simulink model "Slx002_M1_TTRobot"  (R2017b)
settings: Solver=FixedStepAuto  StartTime=0  StopTime=100.0  FixedStep=0.001  RelTol=1e-3
settings Model: Creator=Dell  LastModifiedBy=Dell

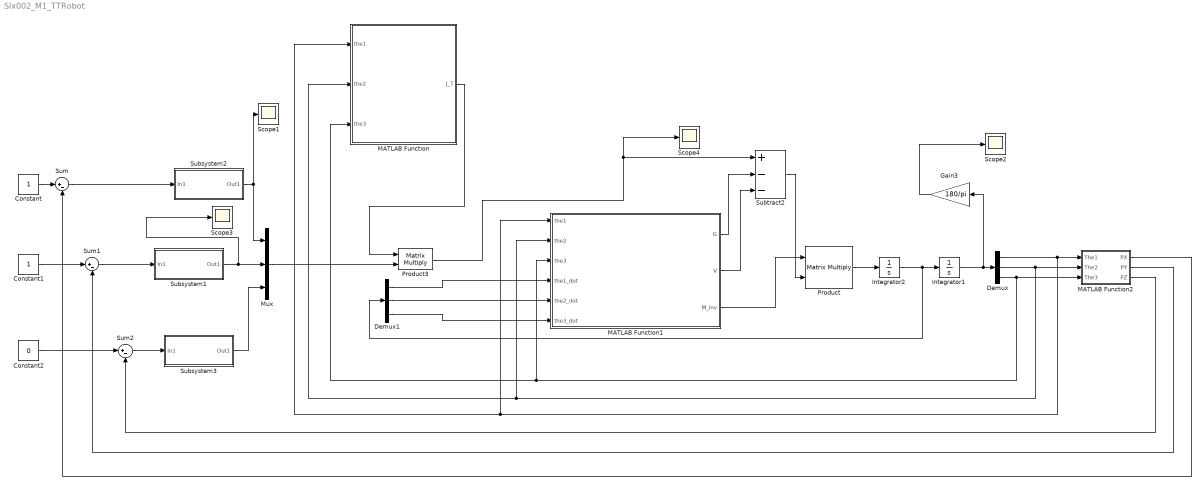
== system Slx002_M1_TTRobot ==
  Constant : Constant
  Constant1 : Constant
  Constant2 : Constant  Value=0
  Demux : Demux  Outputs=3
  Demux1 : Demux  Outputs=3
  Gain3 : Gain  Gain=180/pi
  Integrator1 : Integrator  InitialCondition=[pi/4; 0; 0]
  Integrator2 : Integrator  InitialCondition=[0; 0; 0]
  MATLAB Function : MATLAB Function  TreatAsAtomicUnit=on
  MATLAB Function1 : MATLAB Function  TreatAsAtomicUnit=on
  MATLAB Function2 : MATLAB Function  TreatAsAtomicUnit=on
  Mux : Mux  Inputs=3
  Product : Product  Multiplication=Matrix(*)
  Product3 : Product  Multiplication=Matrix(*)
  Scope{1..4} (4 alike) : Scope
  Subsystem1 : Subsystem  mask{Kp=32, Ki=30, Kd=22}
  Subsystem2 : Subsystem  mask{Kp=30, Ki=12, Kd=20}
  Subsystem3 : Subsystem  mask{Kp=32, Ki=30, Kd=22}
  Subtract2 : Sum  Inputs=+--
  Sum : Sum  Inputs=|+-
  Sum1 : Sum  Inputs=|+-
  Sum2 : Sum  Inputs=|+-
  wires:
  Sum/1 -> Subsystem2/1(In1)
  MATLAB Function2/1(PX) -> Sum/2
  Subsystem1/1(Out1) -> Mux/2, Scope3/1
  MATLAB Function1/2(V) -> Subtract2/3
  Product3/1 -> Scope4/1, Subtract2/1
  Subsystem2/1(Out1) -> Mux/1, Scope1/1
  Mux/1 -> Product3/2
  MATLAB Function2/2(PY) -> Sum1/2
  MATLAB Function/1(J_T) -> Product3/1
  Demux1/1 -> MATLAB Function1/4(the1_dot)
  Demux1/2 -> MATLAB Function1/5(the2_dot)
  MATLAB Function1/1(G) -> Subtract2/2
  Constant1/1 -> Sum1/1
  Sum1/1 -> Subsystem1/1(In1)
  Integrator1/1 -> Demux/1, Gain3/1
  Subtract2/1 -> Product/2
  Demux/2 -> MATLAB Function1/2(the2), MATLAB Function/2(the2), MATLAB Function2/2(The2)
  MATLAB Function1/3(M_inv) -> Product/1
  Integrator2/1 -> Demux1/1, Integrator1/1
  Demux/1 -> MATLAB Function/1(the1), MATLAB Function1/1(the1), MATLAB Function2/1(The1)
  Gain3/1 -> Scope2/1
  Product/1 -> Integrator2/1
  Constant/1 -> Sum/1
  Demux/3 -> MATLAB Function1/3(the3), MATLAB Function/3(the3), MATLAB Function2/3(The3)
  Sum2/1 -> Subsystem3/1(In1)
  Constant2/1 -> Sum2/1
  Subsystem3/1(Out1) -> Mux/3
  MATLAB Function2/3(PZ) -> Sum2/2
  Demux1/3 -> MATLAB Function1/6(the3_dot)

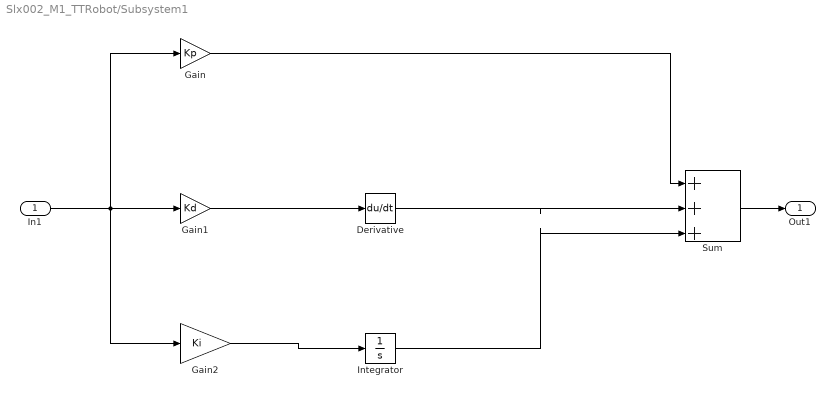
== system Slx002_M1_TTRobot/Subsystem1 ==
  In1 : Inport
  Derivative : Derivative
  Gain : Gain  Gain=Kp
  Gain1 : Gain  Gain=Kd
  Gain2 : Gain  Gain=Ki
  Integrator : Integrator
  Sum : Sum  Inputs=|+++
  Out1 : Outport
  wires:
  Sum/1 -> Out1/1
  Gain/1 -> Sum/1
  Gain1/1 -> Derivative/1
  Derivative/1 -> Sum/2
  Gain2/1 -> Integrator/1
  Integrator/1 -> Sum/3
  In1/1 -> Gain2/1, Gain/1, Gain1/1

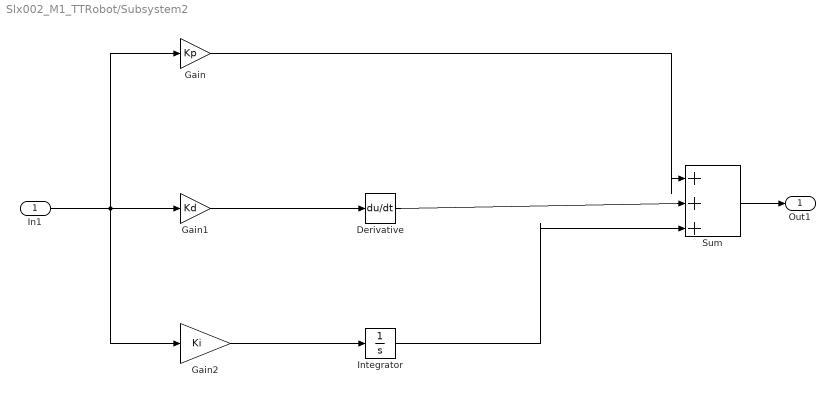
== system Slx002_M1_TTRobot/Subsystem2 ==
  In1 : Inport
  Derivative : Derivative
  Gain : Gain  Gain=Kp
  Gain1 : Gain  Gain=Kd
  Gain2 : Gain  Gain=Ki
  Integrator : Integrator
  Sum : Sum  Inputs=|+++
  Out1 : Outport
  wires:
  Sum/1 -> Out1/1
  Gain/1 -> Sum/1
  Gain1/1 -> Derivative/1
  Derivative/1 -> Sum/2
  Gain2/1 -> Integrator/1
  Integrator/1 -> Sum/3
  In1/1 -> Gain2/1, Gain/1, Gain1/1

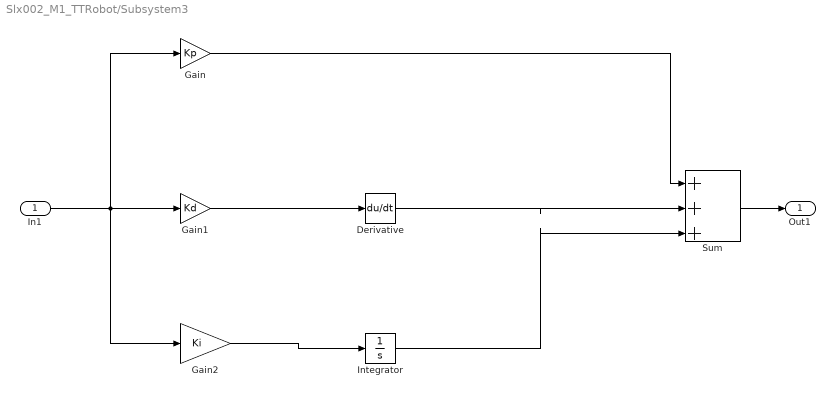
== system Slx002_M1_TTRobot/Subsystem3 ==
  In1 : Inport
  Derivative : Derivative
  Gain : Gain  Gain=Kp
  Gain1 : Gain  Gain=Kd
  Gain2 : Gain  Gain=Ki
  Integrator : Integrator
  Sum : Sum  Inputs=|+++
  Out1 : Outport
  wires:
  Sum/1 -> Out1/1
  Gain/1 -> Sum/1
  Gain1/1 -> Derivative/1
  Derivative/1 -> Sum/2
  Gain2/1 -> Integrator/1
  Integrator/1 -> Sum/3
  In1/1 -> Gain2/1, Gain/1, Gain1/1

== matlab function Slx002_M1_TTRobot/MATLAB Function1 ==
  data: G output; V output; the1 input; the2 input; the3 input; M_inv output; the1_dot input; the2_dot input; the3_dot input
function [G, V, M_inv] = fcn(the1, the2, the3, the1_dot, the2_dot, the3_dot)
d2=1; d5=1; g=9.81; m1=1; m2=1; mEE=1;

c2=cos(the2);
s2=sin(the2);
c3=cos(the3);
s3=sin(the3);
c23=cos(the2 + the3);
s23=sin(the2+the3);
c12 = cos(the1+the2);
s12 = sin(the1+the2);


m11 = 0;
m12 = 0;
m13 = 0;
m21 = 0;
m22 = d2*d2*m2 + d2*d2*mEE + d5*mEE + 2*d2*d5*mEE*c3;
m23 = d5*d5*mEE + d2*d5*mEE*c3;
m31 = 0;
m32 = d5*d5*mEE + d2*d5*mEE*c3;
m33 = d5*d5*mEE;

M = [m11 m12 m13; m21 m22 m23; m31 m32 m33];
M_inv = inv(M);

v1 = 0;
g1 = 0;

v2 = -d2*d5*mEE*s3*the3_dot*the3_dot -2*d2*d5*mEE*s3*the2_dot*the3_dot;
g2 = 0;

v3 = d2*d5*mEE*s3*the2_dot*the2_dot;
g3 = 0;


G = [g1; g2; g3];
V = [v1; v2; v3];

== matlab function Slx002_M1_TTRobot/MATLAB Function ==
  data: the1 input; the2 input; J_T output; the3 input
function J_T  = fcn(the1, the2, the3)
d2=1; d5=1; g=9.81; m1=1; m2=1; mEE=1;
c2=cos(the2);
s2=sin(the2);
c23=cos(the2 + the3);
s23=sin(the2+the3);
c12 = cos(the1+the2);
s12 = sin(the1+the2);

% P_0_EE = [(d5*c23 + d2*c2); (d5*s23 + d2*s2); 0];
J11 = 0;
J12 = -d5*s23 -d2*s2;
J13 = -d5*s23;
J21 = 0;
J22 = d5*c23 + d2*c2;
J23 = d5*c23;
J31 = 0;
J32 = 0;
J33 = 0;
J = [J11 J12 J13;...
     J21 J22 J23;...
     J31 J32 J33];
J_T = [J(1,1) J(2,1) J(3,1);...
       J(1,2) J(2,2) J(3,2);...
       J(1,3) J(2,3) J(3,3)];

== matlab function Slx002_M1_TTRobot/MATLAB Function2 ==
  data: The1 input; PX output; The2 input; PY output; The3 input; PZ output
function [PX, PY, PZ] = fcn(The1, The2, The3)
d2=1; d5=1;
PX = d2*cos(The2) + d5*(cos(The2)*cos(The3) - sin(The2)*sin(The3));
PY = d2*sin(The2) + d5*(cos(The2)*sin(The3) + cos(The3)*sin(The2));
PZ = 0;

%%P = [PX;PY];
